simulink model "Malha_Aberta"  (R2015a)
settings: Solver=FixedStepDiscrete  StartTime=0.0  StopTime=inf  RelTol=1e-3
undefined symbols (not defined in the file): velocidade
libraries: arduinolib x2
settings Model: SimulationMode=external  ExtModeTrigDuration=2  Creator=kelvin  LastModifiedBy=kelvin
settings OptimizationCC: OptimizeModelRefInitCode=on  LifeSpan=1
settings DebuggingCC: UnderspecifiedInitializationDetection=Classic  MergeDetectMultiDrivingBlocksExec=none
settings HardwareCC: ProdBitPerInt=16  ProdBitPerPointer=8  ProdIntDivRoundTo=Zero  ProdEndianess=LittleEndian  ProdWordSize=8  ProdHWDeviceType=Atmel->AVR
settings RTWCC: SystemTargetFile=realtime.tlc  GenerateMakefile=off  TemplateMakefile=realtime.tmf  Description=Run on Target Hardware  RTWVerbose=off
settings ERTTargetCC: CombineOutputUpdateFcns=off  ExtModeTransport=3  ExtModeMexFile=ext_serial_win32_comm_rtt  ExtModeMexArgs=0 1 9600  ERTSrcFileBannerTemplate=realtime_code_template.cgt  ERTHdrFileBannerTemplate=realtime_code_template.cgt  ERTDataSrcFileTemplate=realtime_code_template.cgt  ERTDataHdrFileTemplate=realtime_code_template.cgt  ERTCustomFileTemplate=realtime_file_process.tlc

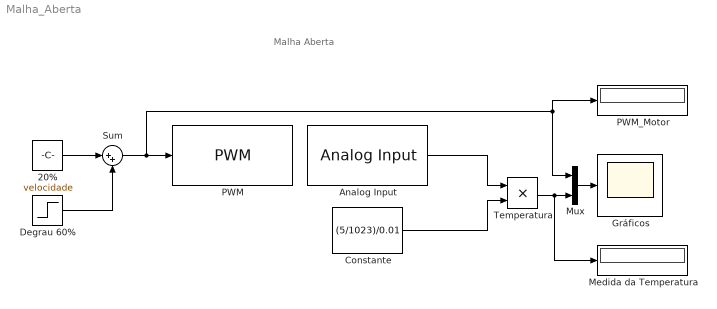
== system Malha_Aberta ==
  note: Malha Aberta
  20% : Constant  Value=velocidade  VectorParams1D=off
  Analog Input : arduinolib/Analog Input  pinNumber=0  sampleTime=0.01  blockPlatform=arduino
  Constante : Constant  Value=(5/1023)/0.01
  Degrau 60% : Step  Time=3000  After=102  SampleTime=0.01
  Gráficos : Scope
      settings: ShowLegends=on  TimeRange=279.0344752239425  YMin=36.25489937023825  YMax=52.67274408772624  SaveName=Dados_tempo_real
  Medida da Temperatura : Display
  Mux : Mux  Inputs=2
  PWM : arduinolib/PWM  pinNumber=9  blockPlatform=arduino
  PWM_Motor : Display
  Sum : Sum  Inputs=|++
  Temperatura : Product
  wires:
  20%/1 -> Sum/1
  Analog Input/1 -> Temperatura/1
  Constante/1 -> Temperatura/2
  Mux/1 -> Gráficos/1
  Temperatura/1 -> Medida da Temperatura/1, Mux/2
  Sum/1 -> PWM_Motor/1, Mux/1, PWM/1
  Degrau 60%/1 -> Sum/2
